simulink model "Model_IPS3"  (R2016a)
settings: Solver=VariableStepAuto  StartTime=0  StopTime=3
values from neighbouring files (symbols this model uses):
  Imrn = 7.4    [parametriAM.m]
  In = 12.7    [parametriAM.m]
  Ismax = In*sqrt(2)    [parametriAM.m]
  J = 0.019    [parametriAM.m]    (also in podatki.m = 0.01)
  Ki_Imr = 1000    [parametriAM.m]
  Ki_tok = 5.0    (= 5)    [parametriAM.m]
  Ki_wr = 1000    [parametriAM.m]
  Kp_Imr = 100    [parametriAM.m]
  Kp_tok = 0.05    [parametriAM.m]
  Kp_wr = 50    [parametriAM.m]
  Lm = 0.0493    [parametriAM.m]    (also in podatki.m = 0.2342)
  Lr = 0.05315    [parametriAM.m]    (also in podatki.m = 0.2449)
  Ls = 0.05315    [parametriAM.m]    (also in podatki.m = 0.2449)
  Lst = sigma*Ls    (= 0.00742111947319)    [parametriAM.m]
  pp = 3    [parametriAM.m]    (also in podatki.m = 2)
  Rs = 0.594    [parametriAM.m]    (also in podatki.m = 3.7)
  sigma = 1 - 1/((1+sigmaR)*(1+sigmaS))    (= 0.13962595434)    [parametriAM.m]
  taufiltra = 1/(2*pi*fcutoff)    (= 1.59154943092e-05)    [parametriAM.m]
  Tr = Lr/Rr    (= 0.0771407837446)    [parametriAM.m]
  Udc = Un*sqrt(2/3*2)    [parametriAM.m]
  Usmax = Udc    [parametriAM.m]
  wb_upper_limit_field_weaking = sqrt((Ls^2+Lst^2)/(2*Lst^2*Ls^2))*Un/Ismax    [parametriAM.m]
  wdod = 2000*2*pi/60    (= 209.439510239)    [parametriAM.m]
libraries: simulink x15
(part 2 of 2)

== system Model_IPS3/Subsystem6/Clarke/ABC_ab1 ==
  A : Inport
  B : Inport  Port=2
  C : Inport  Port=3
  Gain1 : Gain  Gain=2
  Gain2 : Gain
  Gain24 : Gain  Gain=sqrt(3)/3
  Sum11 : Sum
  Terminator : Terminator
  alfa : Outport
  beta : Outport  Port=2
  wires:
  C/1 -> Terminator/1
  Gain1/1 -> Sum11/2
  B/1 -> Gain1/1
  Gain24/1 -> beta/1
  Gain2/1 -> alfa/1
  Sum11/1 -> Gain24/1
  A/1 -> Sum11/1, Gain2/1

== system Model_IPS3/Subsystem6/Inverzni Clarke/ab_ABC ==
  alfa : Inport
  beta : Inport  Port=2
  Gain1 : Gain
  Gain2 : Gain  Gain=-0.5
  Gain25 : Gain  Gain=sqrt(3)/2
  Gain3 : Gain  Gain=sqrt(3)/2
  Gain4 : Gain  Gain=0.5
  Sum10 : Sum
  Sum11 : Sum  Inputs=--
  A : Outport
  B : Outport  Port=2
  C : Outport  Port=3
  wires:
  Gain3/1 -> Sum11/2
  beta/1 -> Gain25/1, Gain3/1
  Gain4/1 -> Sum11/1
  Gain25/1 -> Sum10/2
  Gain2/1 -> Sum10/1
  alfa/1 -> Gain1/1, Gain2/1, Gain4/1
  Gain1/1 -> A/1
  Sum10/1 -> B/1
  Sum11/1 -> C/1
